simulink model "one_tank_laminar"  (R2020a)
settings: Solver=VariableStepAuto  StartTime=0.0  StopTime=time  RelTol=1e-3
undefined symbols (not defined in the file): qin, resistance, tao
settings Model: Creator=jilve  LastModifiedBy=jilve

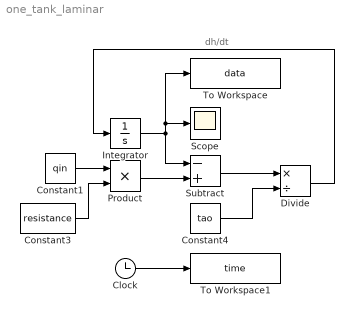
== system one_tank_laminar ==
  note: dh/dt
  Clock : Clock
      settings: Decimation=time
  Constant1 : Constant  Value=qin
  Constant3 : Constant  Value=resistance
  Constant4 : Constant  Value=tao
  Divide : Product  Inputs=*/
  Integrator : Integrator
  Product : Product
  Scope : Scope
  Subtract : Sum  Inputs=-+
  To Workspace : ToWorkspace  VariableName=data  SampleTime=-1
  To Workspace1 : ToWorkspace  VariableName=time  SampleTime=-1
  wires:
  Constant1/1 -> Product/1
  Constant3/1 -> Product/2
  Product/1 -> Subtract/2
  Constant4/1 -> Divide/2
  Subtract/1 -> Divide/1
  Divide/1 -> Integrator/1
  Integrator/1 -> To Workspace/1, Scope/1, Subtract/1
  Clock/1 -> To Workspace1/1
